simulink model "Model_4"  (R2020b)
settings: Solver=VariableStepAuto  StartTime=0.0  StopTime=2  RelTol=1e-3
values from neighbouring files (symbols this model uses):
  b = 3.5077E-6    [Motor_position_data.sldd]    (also in Variables.m = 3.5077e-06)
  J = 3.2284E-6    [Motor_position_data.sldd]    (also in Variables.m = 3.2284e-06)
  K = 0.0274    [Variables.m]
  L = 2.75E-6    [Motor_position_data.sldd]    (also in Variables.m = 2.75e-06)
  R = 4.0    [Motor_position_data.sldd]    (also in Variables.m = 4)
settings Model: DataDictionary=Data_Dictionary.sldd  Creator=samar  LastModifiedBy=samar

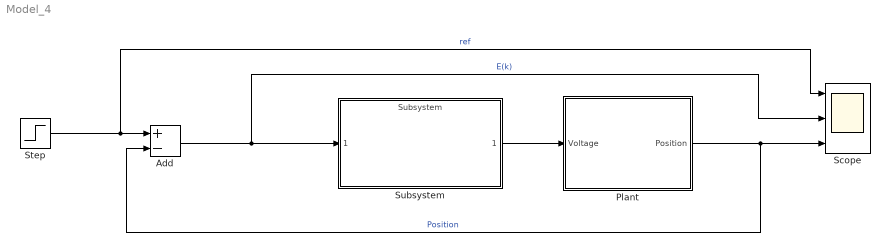
== system Model_4 ==
  Add : Sum  Inputs=+-
  Plant : Subsystem
  Scope : Scope  NumInputPorts=3
  Step : Step  SampleTime=0
  Subsystem : ModelReference  ModelNameDialog=Subsystem  SimulationMode=Normal  ModelReferenceVersion=1.7  mask{Kp=18842.98, Ki=12396450.71, Kd=6.98}
  wires:
  Plant/1(Position) -> Add/2, Scope/3  "Position"
  Subsystem/1 -> Plant/1(Voltage)
  Step/1 -> Scope/1, Add/1  "ref"
  Add/1 -> Subsystem/1, Scope/2  "E(k)"

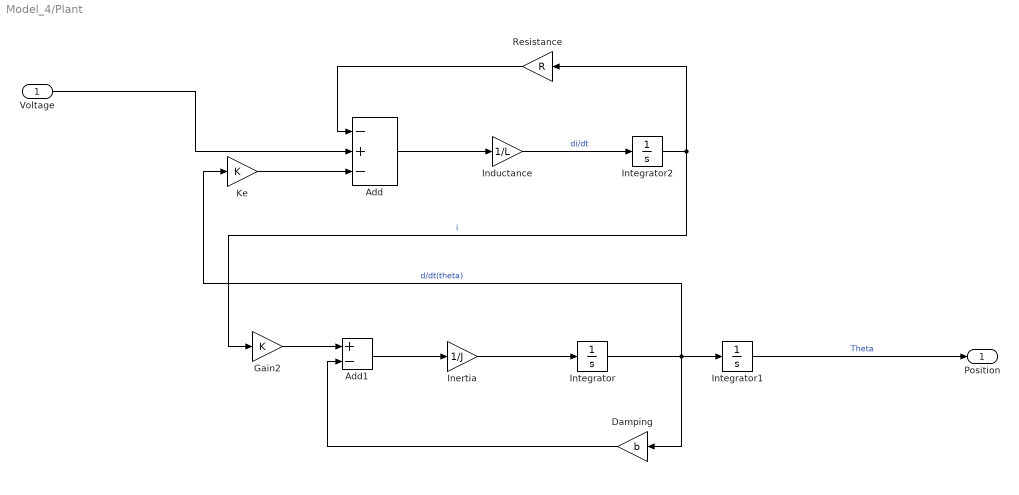
== system Model_4/Plant ==
  Voltage : Inport
  Add : Sum  Inputs=-+-
  Add1 : Sum  Inputs=+-
  Damping : Gain  Gain=b
  Gain2 : Gain  Gain=K
  Inductance : Gain  Gain=1/L
  Inertia : Gain  Gain=1/J
  Integrator : Integrator
  Integrator1 : Integrator
  Integrator2 : Integrator
  Ke : Gain  Gain=K
  Resistance : Gain  Gain=R
  Position : Outport
  wires:
  Damping/1 -> Add1/2
  Inductance/1 -> Integrator2/1  "di/dt"
  Inertia/1 -> Integrator/1
  Integrator2/1 -> Gain2/1, Resistance/1  "i"
  Ke/1 -> Add/3
  Integrator/1 -> Ke/1, Integrator1/1, Damping/1  "d/dt(theta)"
  Add1/1 -> Inertia/1
  Resistance/1 -> Add/1
  Add/1 -> Inductance/1
  Gain2/1 -> Add1/1
  Voltage/1 -> Add/2
  Integrator1/1 -> Position/1  "Theta"
